simulink model "vanderpol"  (R2023a)
settings: Solver=ode1  StartTime=0.0  StopTime=1000  FixedStep=0.002  RelTol=1e-3
values from neighbouring files (symbols this model uses):
  cycleGain = 0.2    [simulate_hover.m]    (also in temp.m = 1)
libraries: simulink_extras x2
settings Model: Creator=Jacob  LastModifiedBy=Jacob
settings DataIOCC: ReturnWorkspaceOutputs=off

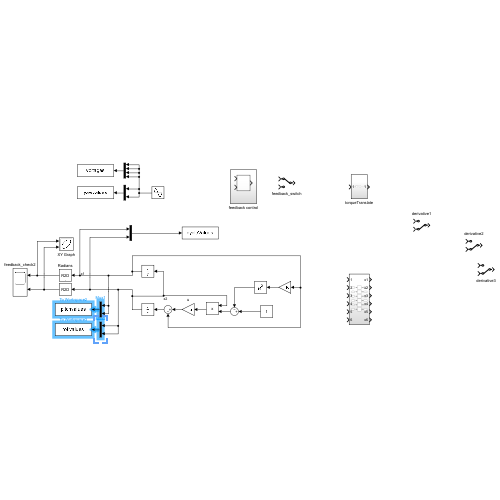
[thumbnail: Simulink's stored preview of the top-level diagram]
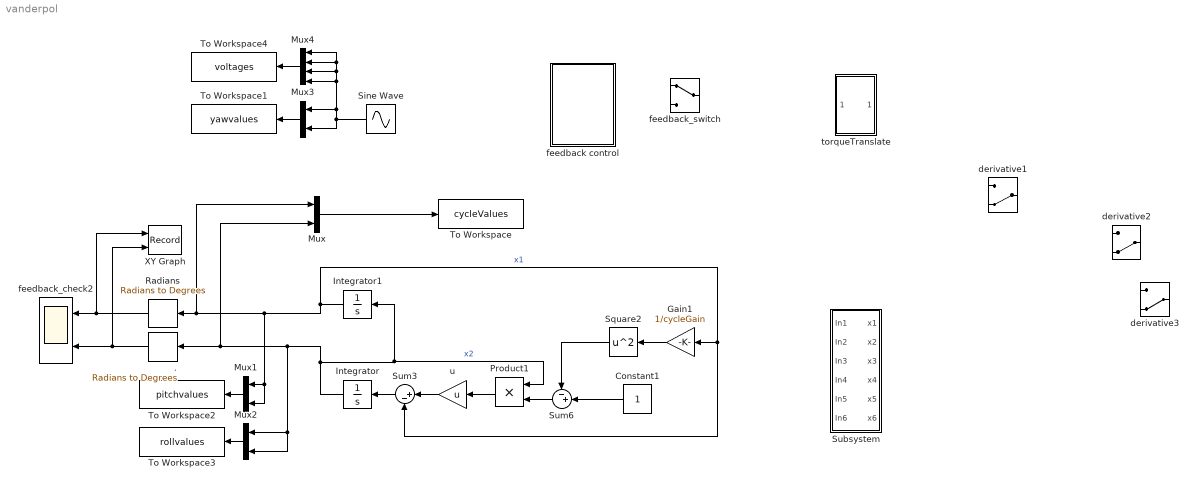
== system vanderpol ==
  . : simulink_extras/Transformations/Radians to Degrees
  Constant1 : Constant
  Gain1 : Gain  Gain=1/cycleGain
  Integrator : Integrator  InitialCondition=0.1
  Integrator1 : Integrator  InitialCondition=0.1
  Mux{,1..3} (4 alike) : Mux  Inputs=2
  Mux4 : Mux
  Product1 : Product
  Radians : simulink_extras/Transformations/Radians to Degrees
  Sine Wave : Sin  SampleTime=0
  Square2 : Math  Operator=square
  Subsystem : Subsystem
  Sum3 : Sum  Inputs=|+-
  Sum6 : Sum  Inputs=-+|
  To Workspace : ToWorkspace  VariableName=cycleValues  SampleTime=-1
  To Workspace1 : ToWorkspace  VariableName=yawvalues  SampleTime=-1
  To Workspace2 : ToWorkspace  VariableName=pitchvalues  SampleTime=-1
  To Workspace3 : ToWorkspace  VariableName=rollvalues  SampleTime=-1
  To Workspace4 : ToWorkspace  VariableName=voltages  SampleTime=-1
  XY Graph : Record  FileSettingsInternal="{\"entries\":[{\"content\":{\"excelSettings\":{\"content\":{},\"type\":\"Streamout.ExcelSettings\"}},\"type\":\"Streamout.FileSettingStorage\",\"uuid\":\"\"}],\"packageUris\":[\"http:\\/\\/schema.mathworks.com\\/mf0\\/streamout_blocks\\/R2020a\"],\"version\":\"1.0\"}"  Layout=[1 1]  SignalsInternal="{\"entries\":[{\"content\":{\"signals\":[{\"content\":{\"blockPath\":[],\"dimensions\":[1],\"domain\":\"\",\"lineColor\":\"#a2142f\",\"plots\":[1],\"port\":1,\"sid\":[\"\"],\"signalID\":12892,\"signalName\":\"Radians\"},\"type\":\"RecordBlkView.Signal\",\"uuid\":\"\"},{\"content\":{\"blockPath\":[],\"dimensions\":[1],\"domain\":\"\",\"lineColor\":\"#139fff\",\"plots\":[1],\"port\":2,\"sid\":[\"\"],\"signalID\":12896,\"signalName\":\".\"},\"type\":\"RecordBlkView.Signal\",\"uuid\":\"\"}]},\"type\":\"RecordBlkView.InputSignals\",\"uuid\":\"\"}],\"packageUris\":[\"http:\\/\\/schema.mathworks.com\\/mf0\\/streamout_blocks\\/R2020a\"],\"version\":\"1.0\"}"  VisualizationBindings="{\"xyplotplugin\":{\"info\":[{\"series\":[{\"bindingParametersList\":[{\"parameter\":\"Y-Axis\",\"signalID\":12896,\"signalName\":\".\"},{\"parameter\":\"X-Axis\",\"signalID\":12892,\"signalName\":\"Radians\"}],\"seriesID\":12475}],\"subplotID\":1}]}}"  CompatibilityTag=XY
  derivative1 : ManualSwitch  CurrentSetting=0
  derivative2 : ManualSwitch  CurrentSetting=0
  derivative3 : ManualSwitch  CurrentSetting=0
  feedback control : Subsystem
  feedback_check2 : Scope  NumInputPorts=2
  feedback_switch : ManualSwitch
  torqueTranslate : Subsystem
  u : Gain  Gain=u
  wires:
  Integrator1/1 -> Mux/1, Radians/1, Mux1/1, Mux1/2, Sum3/2, Gain1/1  "x1"
  Integrator/1 -> Mux2/2, Mux2/1, Mux/2, ./1, Product1/1, Integrator1/1  "x2"
  Sum3/1 -> Integrator/1
  Sum6/1 -> Product1/2
  Product1/1 -> u/1
  u/1 -> Sum3/1
  Square2/1 -> Sum6/1
  Constant1/1 -> Sum6/2
  ./1 -> XY Graph/2, feedback_check2/2
  Radians/1 -> XY Graph/1, feedback_check2/1
  Gain1/1 -> Square2/1
  Mux/1 -> To Workspace/1
  Mux1/1 -> To Workspace2/1
  Mux2/1 -> To Workspace3/1
  Mux3/1 -> To Workspace1/1
  Mux4/1 -> To Workspace4/1
  Sine Wave/1 -> Mux4/4, Mux4/3, Mux4/2, Mux4/1, Mux3/1, Mux3/2

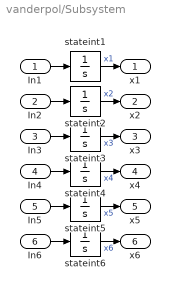
== system vanderpol/Subsystem ==
  In1 : Inport
  In2 : Inport  Port=2
  In3 : Inport  Port=3
  In4 : Inport  Port=4
  In5 : Inport  Port=5
  In6 : Inport  Port=6
  stateint{1..6} (6 alike) : Integrator
  x1 : Outport
  x2 : Outport  Port=2
  x3 : Outport  Port=3
  x4 : Outport  Port=4
  x5 : Outport  Port=5
  x6 : Outport  Port=6
  wires:
  In3/1 -> stateint3/1
  stateint2/1 -> x2/1  "x2"
  stateint5/1 -> x5/1  "x5"
  In2/1 -> stateint2/1
  stateint6/1 -> x6/1  "x6"
  In6/1 -> stateint6/1
  stateint3/1 -> x3/1  "x3"
  In4/1 -> stateint4/1
  stateint4/1 -> x4/1  "x4"
  In5/1 -> stateint5/1
  In1/1 -> stateint1/1
  stateint1/1 -> x1/1  "x1"

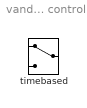
== system vanderpol/feedback control ==
  timebased : ManualSwitch

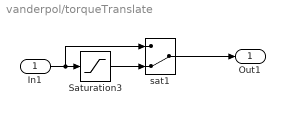
== system vanderpol/torqueTranslate ==
  In1 : Inport
  Saturation3 : Saturate  UpperLimit=24  LowerLimit=-24
  sat1 : ManualSwitch  CurrentSetting=0
  Out1 : Outport
  wires:
  In1/1 -> sat1/1, Saturation3/1
  Saturation3/1 -> sat1/2
  sat1/1 -> Out1/1
